simulink model "TRLQR"  (R2025a)
settings: Solver=VariableStepAuto  StartTime=0.0  StopTime=10.0  RelTol=1e-3
undefined symbols (not defined in the file): L, start, theta0
settings Model: Creator=mwali  LastModifiedBy=mwali

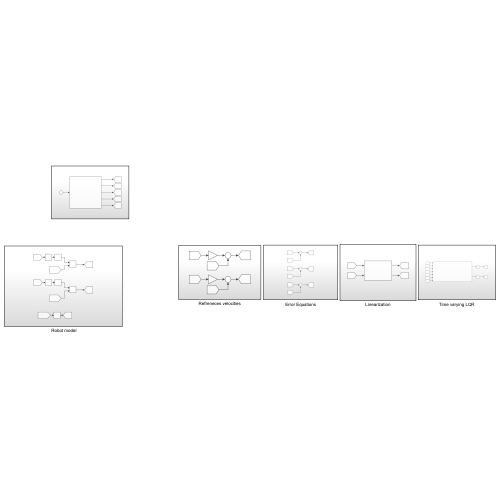
[thumbnail: Simulink's stored preview of the top-level diagram]
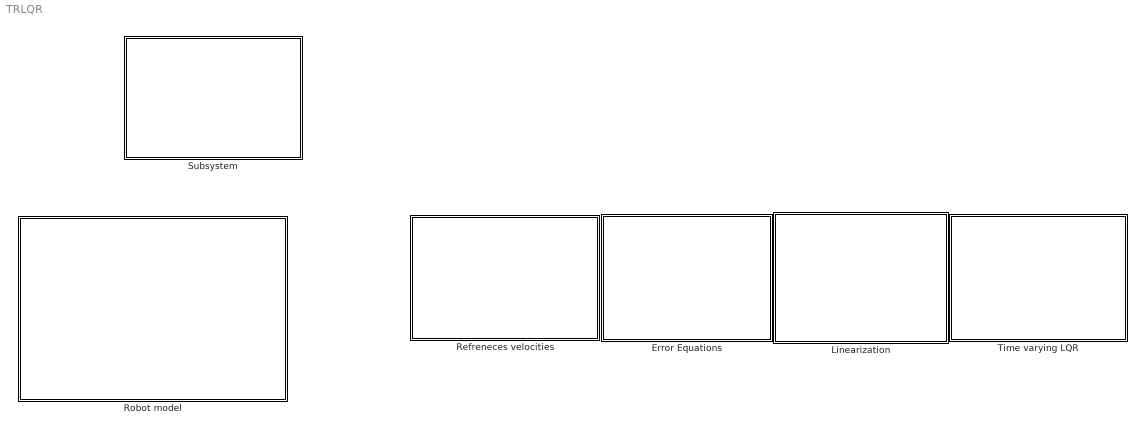
== system TRLQR ==
  " Robot model" : Subsystem
  Error Equations : Subsystem
  Linearization : Subsystem
  Refreneces velocities : Subsystem
  Subsystem : Subsystem
  Time varying LQR : Subsystem

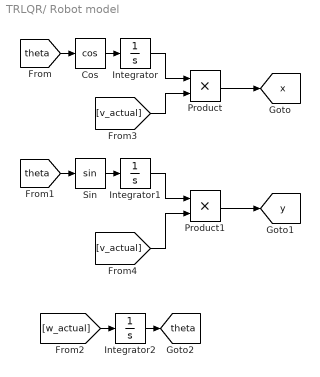
== system TRLQR/ Robot model ==
  Cos : Trigonometry  Operator=cos
  Integrator : Integrator  InitialCondition=start(1)
  Integrator1 : Integrator  InitialCondition=start(2)
  Integrator2 : Integrator  InitialCondition=theta0
  Product : Product
  Product1 : Product
  Sin : Trigonometry
  tag scope: theta=global, x=global, y=global
  wires:
  Sin/1 -> Integrator1/1
  [theta] -> Sin/1
  Cos/1 -> Integrator/1
  Integrator2/1 -> [theta]
  [theta] -> Cos/1
  [w_actual] -> Integrator2/1
  Integrator/1 -> Product/1
  [v_actual] -> Product/2
  Product/1 -> [x]
  Integrator1/1 -> Product1/1
  [v_actual] -> Product1/2
  Product1/1 -> [y]

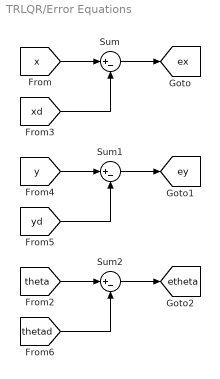
== system TRLQR/Error Equations ==
  Sum : Sum  Inputs=|+-
  Sum1 : Sum  Inputs=|+-
  Sum2 : Sum  Inputs=|+-
  tag scope: etheta=global, ex=global, ey=global
  wires:
  [y] -> Sum1/1
  Sum/1 -> [ex]
  [x] -> Sum/1
  [yd] -> Sum1/2
  Sum1/1 -> [ey]
  [theta] -> Sum2/1
  [thetad] -> Sum2/2
  Sum2/1 -> [etheta]
  [xd] -> Sum/2

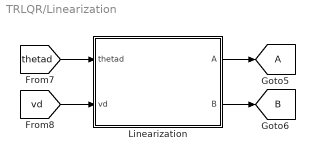
== system TRLQR/Linearization ==
  Goto5 : Goto  TagVisibility=global
  "Linearization " : MATLAB Function  TreatAsAtomicUnit=on
  tag scope: B=global
  wires:
  "Linearization "/1(A) -> Goto5/1
  "Linearization "/2(B) -> [B]
  [vd] -> "Linearization "/2(vd)
  [thetad] -> "Linearization "/1(thetad)

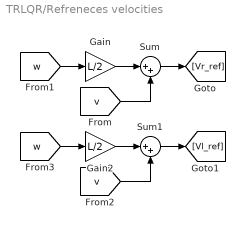
== system TRLQR/Refreneces velocities ==
  Gain : Gain  Gain=L/2
  Gain2 : Gain  Gain=L/2
  Sum : Sum  Inputs=|++
  Sum1 : Sum  Inputs=|++
  wires:
  [v] -> Sum/2
  Sum/1 -> [Vr_ref]
  Gain/1 -> Sum/1
  [w] -> Gain/1
  Gain2/1 -> Sum1/1
  [v] -> Sum1/2
  [w] -> Gain2/1
  Sum1/1 -> [Vl_ref]

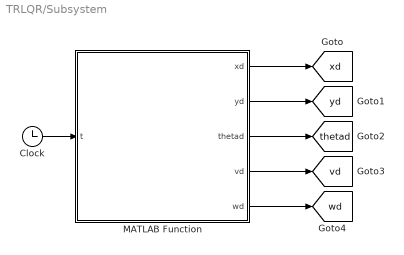
== system TRLQR/Subsystem ==
  Clock : Clock
  MATLAB Function : MATLAB Function  TreatAsAtomicUnit=on
  tag scope: thetad=global, vd=global, wd=global, xd=global, yd=global
  wires:
  Clock/1 -> MATLAB Function/1(t)
  MATLAB Function/1(xd) -> [xd]
  MATLAB Function/2(yd) -> [yd]
  MATLAB Function/3(thetad) -> [thetad]
  MATLAB Function/4(vd) -> [vd]
  MATLAB Function/5(wd) -> [wd]

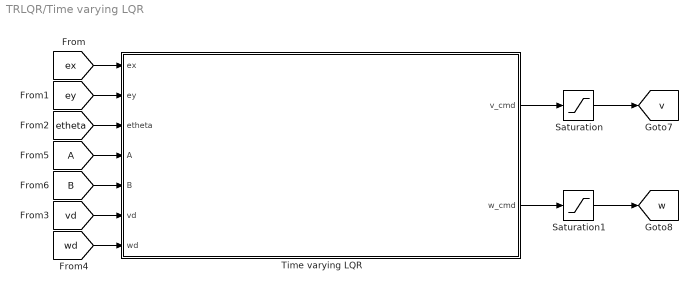
== system TRLQR/Time varying LQR ==
  From5 : From
  Saturation : Saturate  UpperLimit=0.6  LowerLimit=0
  Saturation1 : Saturate  UpperLimit=2  LowerLimit=-2
  Time varying LQR : MATLAB Function  TreatAsAtomicUnit=on
  tag scope: v=global, w=global
  wires:
  Time varying LQR/2(w_cmd) -> Saturation1/1
  [ex] -> Time varying LQR/1(ex)
  Saturation1/1 -> [w]
  [ey] -> Time varying LQR/2(ey)
  From5/1 -> Time varying LQR/4(A)
  [etheta] -> Time varying LQR/3(etheta)
  Time varying LQR/1(v_cmd) -> Saturation/1
  [vd] -> Time varying LQR/6(vd)
  [wd] -> Time varying LQR/7(wd)
  [B] -> Time varying LQR/5(B)
  Saturation/1 -> [v]

== matlab function TRLQR/Linearization/Linearization  ==
  data: thetad input; A output; vd input; B output
function [A,B] = linearizeRobot(thetad,vd)

A = [0 0 -vd*sin(thetad);
     0 0  vd*cos(thetad);
     0 0  0];

B = [cos(thetad) 0;
     sin(thetad) 0;
     0           1];

== matlab function TRLQR/Subsystem/MATLAB Function ==
  data: t input; xd output; yd output; thetad output; vd output; wd output
function [xd, yd, thetad, vd, wd] = referenceGenerator(t)

P = evalin('base','P');
theta_ref = evalin('base','theta_ref');
vd_ref = evalin('base','vd_ref');
wd_ref = evalin('base','wd_ref');
Ts_ref = evalin('base','Ts_ref');

idx = floor(t / Ts_ref) + 1;

if idx > size(P,1)
    idx = size(P,1);
end

xd = P(idx,1);
yd = P(idx,2);
thetad = theta_ref(idx);
vd = vd_ref(idx);
wd = wd_ref(idx);

== matlab function TRLQR/Time varying LQR/Time varying LQR ==
  data: ex input; v_cmd output; ey input; etheta input; A input; B input; vd input; wd input; w_cmd output
function [v_cmd, w_cmd] = tvlqrControl(ex, ey, etheta, A, B, vd, wd)

Q = diag([10 10 5]);
R = diag([1 1]);

K = lqr(A, B, Q, R);

e = [ex; ey; etheta];
u_corr = -K * e;

v_cmd = vd + u_corr(1);
w_cmd = wd + u_corr(2);
